simulink model "PubIfDecisionLM_MDL"  (R2020b)
settings: configuration reference "DspaceConfig" (kept outside this file)
PostLoadFcn:
  | if any(exist('dsrtsu_mdlpostloadfcn', 'file') ~= 0), dsrtsu_mdlpostloadfcn('Execute', bdroot); end
InitFcn:
  | , if any(exist('dsmpb_private', 'file') ~= 0), dsmpb_private('dsmpb_mdlclblib', 'Init', bdroot); end,
undefined symbols (not defined in the file or in its folder): OFM_OBJ_FUSIONTYPE_E, OFM_OBJ_MOVINGSTATE_E, OFM_OBJ_ORIENTATION_E, OFM_OBJ_TYPE_E, P_LM_Cyc, P_LM_EMLHistKapRcdBufSize, P_LM_EMLHistTrajBaseDis, P_LM_EMLHistTrajPNum, P_LM_EMLKapCorrMaxThre, P_LM_EMLMinKapThre, P_LM_EMLPathDisDiffThre, P_LM_EMLQuaFiltPar, P_LM_EMLTurnActKapThre, P_LM_EMLValidQuaThre, P_LM_FntPath1Disgap, P_LM_FntPath1MinDis, P_LM_FntPath1Timegap, P_LM_FntPath2Disgap, P_LM_FntPath2MinDis, P_LM_FntPath2Timegap, P_LM_FntPath3Disgap, P_LM_FntPath3MinDis, P_LM_FntPath3Timegap, P_LM_FusBLParFiltP, P_LM_FusEVDifC2Thre, P_LM_FusEVOPath1AllVSLDisThre, P_LM_FusEVOPath1AllVSLLostNumThre, P_LM_FusEVOPath1AllVSLQuaThre, P_LM_FusEVOPath1OTLFacNLC, P_LM_FusOTLQuaThre, P_LM_FusOTLSW, P_LM_FusParC0Index, P_LM_FusParC1Index, P_LM_FusParC2Index, P_LM_FusParC3Index, P_LM_FusVSLQuaThre, P_LM_FusVSLSW, P_LM_FusVSLValidSteerWheerAngThre, P_LM_FusVSLValidVxvThre, P_LM_LaneWidth, P_LM_OTLBufTPInfoEvaFactor, P_LM_OTLObjNum, P_LM_OTLObjSelectAgeThre, P_LM_OTLObjSelectDxAssessVx, P_LM_OTLObjSelectDxThre, P_LM_OTLObjSelectVxThre, P_LM_OTLObjSelectVyAssessDx, P_LM_OTLObjSelectVyThre, P_LM_OTLTrajPntBaseDis, P_LM_OTLTrajStdThre, P_LM_VSLAvailLineNum, P_LM_VSLBLSDiffThre, P_LM_VSLBLSDisRatio, P_LM_VSLFusBLParFiltP_C1, P_LM_VSLFusBLParFiltP_C2, P_LM_VSLFusBLParFiltP_C3, P_LM_VSLFusBLParFiltP_Quality, P_LM_VSLHistTrajBaseDis, P_LM_VSLHistTrajPNum, P_LM_VSLLCC0diff ... (+18)
libraries: simulink x145, LM_LIB x43
(part 18 of 24)

== system PubIfDecisionLM_MDL/Subsystem2/LM_OTL/LM_OTL_MovObjTrajRecord3/LM_OTL_MovObjSelc/LM_OTL_MovObjInterestedSelc/LM_OTL_ObjSelcIndexCheck/RigObj1Check/If Action Subsystem1 ==
  RigObj1CheckInfo : Inport
  LM_OTL_MovObjValid : Inport  Port=2
  Object_DX : Inport  Port=3
  Action Port : ActionPort  ActionPortLabel=else
  Compare To Constant1 : simulink/Logic and Bit Operations/Compare To Constant  relop=<=  const=-1.45  OutDataTypeStr=boolean
  Compare To Constant2 : simulink/Logic and Bit Operations/Compare To Constant  relop=>  const=-6  OutDataTypeStr=boolean
  Constant : Constant  Value=0  OutDataTypeStr=int32
  Logical Operator : Logic  AllPortsSameDT=off  OutDataTypeStr=boolean
  Logical Operator1 : Logic  AllPortsSameDT=off  OutDataTypeStr=boolean
  Multiport Switch : MultiPortSwitch  Inputs=1
  Multiport Switch1 : MultiPortSwitch  Inputs=1
  Switch : Switch  Criteria=u2 > Threshold
  LM_OTLRigObj1Index : Outport
  wires:
  Logical Operator1/1 -> Logical Operator/2
  Logical Operator/1 -> Switch/2
  Multiport Switch1/1 -> Compare To Constant2/1, Compare To Constant1/1
  Compare To Constant1/1 -> Logical Operator1/1
  Compare To Constant2/1 -> Logical Operator1/2
  Object_DX/1 -> Multiport Switch1/2
  LM_OTL_MovObjValid/1 -> Multiport Switch/2
  RigObj1CheckInfo/1 -> Multiport Switch1/1, Multiport Switch/1, Switch/1
  Switch/1 -> LM_OTLRigObj1Index/1
  Constant/1 -> Switch/3
  Multiport Switch/1 -> Logical Operator/1

== system PubIfDecisionLM_MDL/Subsystem2/LM_OTL/LM_OTL_MovObjTrajRecord3/LM_OTL_MovObjSelc/LM_OTL_MovObjInterestedSelc/LM_OTL_ObjSelcIndexCheck/RigObj2Check/If Action Subsystem ==
  Action Port : ActionPort  ActionPortLabel=if(u1 == 0)
  Constant : Constant  Value=0  OutDataTypeStr=int32
  LM_OTLLeObj1Index : Outport
  wires:
  Constant/1 -> LM_OTLLeObj1Index/1

== system PubIfDecisionLM_MDL/Subsystem2/LM_OTL/LM_OTL_MovObjTrajRecord3/LM_OTL_MovObjSelc/LM_OTL_MovObjInterestedSelc/LM_OTL_ObjSelcIndexCheck/RigObj2Check/If Action Subsystem1 ==
  RigObj2CheckInfo : Inport
  LM_OTL_MovObjValid : Inport  Port=2
  Object_DX : Inport  Port=3
  Action Port : ActionPort  ActionPortLabel=else
  Compare To Constant1 : simulink/Logic and Bit Operations/Compare To Constant  relop=<=  const=-2  OutDataTypeStr=boolean
  Compare To Constant2 : simulink/Logic and Bit Operations/Compare To Constant  relop=>  const=-6  OutDataTypeStr=boolean
  Constant : Constant  Value=0  OutDataTypeStr=int32
  Logical Operator : Logic  AllPortsSameDT=off  OutDataTypeStr=boolean
  Logical Operator1 : Logic  AllPortsSameDT=off  OutDataTypeStr=boolean
  Multiport Switch : MultiPortSwitch  Inputs=1
  Multiport Switch1 : MultiPortSwitch  Inputs=1
  Switch : Switch  Criteria=u2 > Threshold
  LM_OTLRigObj2Index : Outport
  wires:
  Logical Operator1/1 -> Logical Operator/2
  Logical Operator/1 -> Switch/2
  Multiport Switch1/1 -> Compare To Constant2/1, Compare To Constant1/1
  Compare To Constant1/1 -> Logical Operator1/1
  Compare To Constant2/1 -> Logical Operator1/2
  Object_DX/1 -> Multiport Switch1/2
  LM_OTL_MovObjValid/1 -> Multiport Switch/2
  RigObj2CheckInfo/1 -> Multiport Switch1/1, Multiport Switch/1, Switch/1
  Switch/1 -> LM_OTLRigObj2Index/1
  Constant/1 -> Switch/3
  Multiport Switch/1 -> Logical Operator/1

== system PubIfDecisionLM_MDL/Subsystem2/LM_OTL/LM_OTL_MovObjTrajRecord3/LM_OTL_MovObjSelc/Subsystem3/LM_OTL_MovObjSelect/LM_OTL_ExistProbAssess/MultiRader ==
  Action Port : ActionPort  ActionPortLabel=elseif((u1==6|u1==10|u1==12|u1==14))
  Constant : Constant  Value=0.5
  Out1 : Outport
  wires:
  Constant/1 -> Out1/1

== system PubIfDecisionLM_MDL/Subsystem2/LM_OTL/LM_OTL_MovObjTrajRecord3/LM_OTL_MovObjSelc/Subsystem3/LM_OTL_MovObjSelect/LM_OTL_ExistProbAssess/Rader&Video ==
  Action Port : ActionPort  ActionPortLabel=elseif((u1==3|u1==5|u1==7|u1==9|u1==11|u1==13|u1==15))
  Constant : Constant  Value=0.4
  Out1 : Outport
  wires:
  Constant/1 -> Out1/1

== system PubIfDecisionLM_MDL/Subsystem2/LM_OTL/LM_OTL_MovObjTrajRecord3/LM_OTL_MovObjSelc/Subsystem3/LM_OTL_MovObjSelect/LM_OTL_ExistProbAssess/Rader&Video1 ==
  Action Port : ActionPort  ActionPortLabel=else
  Constant : Constant  Value=0
  Out1 : Outport
  wires:
  Constant/1 -> Out1/1

== system PubIfDecisionLM_MDL/Subsystem2/LM_OTL/LM_OTL_MovObjTrajRecord3/LM_OTL_MovObjSelc/Subsystem3/LM_OTL_MovObjSelect/LM_OTL_ExistProbAssess/SingleRader ==
  Action Port : ActionPort  ActionPortLabel=if(u1==2|u1==4|u1==8)
  Constant : Constant  Value=0.6
  Out1 : Outport
  wires:
  Constant/1 -> Out1/1

== system PubIfDecisionLM_MDL/Subsystem2/LM_OTL/LM_OTL_MovObjTrajRecord3/LM_OTL_ObjStoreInfoCalc/LM_OTL_BufLe1InfoUpdate1/LM_OTL_BufLe1StoreInfoCalc/LM_OTL_ObjSICCurLeObj1InBufLe1/LM_OTL_BufL1DxInfo ==
  LM_OTLCurLeLaObj1Dx : Inport
  LM_OTLCurLeLaObj1RcdFlg : Inport  Port=2
  Constant : Constant  Value=0  OutDataTypeStr=single
  Switch4 : Switch  Criteria=u2 ~= 0
  LM_OTLBufL1Objdx : Outport
  wires:
  LM_OTLCurLeLaObj1Dx/1 -> Switch4/1
  LM_OTLCurLeLaObj1RcdFlg/1 -> Switch4/2
  Switch4/1 -> LM_OTLBufL1Objdx/1  "LM_OTLBufL1Objdx"
  Constant/1 -> Switch4/3

== system PubIfDecisionLM_MDL/Subsystem2/LM_OTL/LM_OTL_MovObjTrajRecord3/LM_OTL_ObjStoreInfoCalc/LM_OTL_BufLe1InfoUpdate1/LM_OTL_BufLe1StoreInfoCalc/LM_OTL_ObjSICCurLeObj1InBufLe1/LM_OTL_BufL1DyInfo ==
  LM_OTLCurLeLaObj1Dy : Inport
  LM_OTLCurLeLaObj1RcdFlg : Inport  Port=2
  Constant : Constant  Value=0  OutDataTypeStr=single
  Switch4 : Switch  Criteria=u2 ~= 0
  LM_OTLBufL1ObjDy : Outport
  wires:
  Constant/1 -> Switch4/3
  Switch4/1 -> LM_OTLBufL1ObjDy/1  "LM_OTLBufL1ObjDy"
  LM_OTLCurLeLaObj1Dy/1 -> Switch4/1
  LM_OTLCurLeLaObj1RcdFlg/1 -> Switch4/2

== system PubIfDecisionLM_MDL/Subsystem2/LM_OTL/LM_OTL_MovObjTrajRecord3/LM_OTL_ObjStoreInfoCalc/LM_OTL_BufLe1InfoUpdate1/LM_OTL_BufLe1StoreInfoCalc/LM_OTL_ObjSICCurLeObj1InBufLe1/LM_OTL_BufL1EPInfo ==
  note: P_LM_OTLTPNum
  LM_OTLCurLeLaObj1RcdFlg : Inport
  LM_OTLBufL1EPPosK1 : Inport  Port=2
  Add : Sum
  Constant : Constant  OutDataTypeStr=uint8
  Constant1 : Constant  Value=80  OutDataTypeStr=uint8
  Constant2 : Constant  OutDataTypeStr=uint8
  Relational Operator : RelationalOperator  Operator=>  OutDataTypeStr=boolean  RndMeth=Simplest
  Switch1 : Switch  Criteria=u2 ~= 0
  Switch4 : Switch  Criteria=u2 ~= 0
  LM_OTLBufL1EPPos : Outport
  wires:
  Constant/1 -> Add/2
  LM_OTLCurLeLaObj1RcdFlg/1 -> Switch4/2
  LM_OTLBufL1EPPosK1/1 -> Switch4/3, Add/1
  Switch4/1 -> LM_OTLBufL1EPPos/1  "LM_OTLBufL1EPPos"
  Switch1/1 -> Switch4/1
  Relational Operator/1 -> Switch1/2
  Add/1 -> Switch1/3, Relational Operator/1
  Constant1/1 -> Relational Operator/2
  Constant2/1 -> Switch1/1

== system PubIfDecisionLM_MDL/Subsystem2/LM_OTL/LM_OTL_MovObjTrajRecord3/LM_OTL_ObjStoreInfoCalc/LM_OTL_BufLe1InfoUpdate1/LM_OTL_BufLe1StoreInfoCalc/LM_OTL_ObjSICCurLeObj1InBufLe1/LM_OTL_BufL1IDInfo ==
  LM_OTLCurLeLaObj1ID : Inport
  Signal Conversion : SignalConversion  OverrideOpt=off
  LM_OTLBufL1ObjID : Outport
  wires:
  LM_OTLCurLeLaObj1ID/1 -> Signal Conversion/1
  Signal Conversion/1 -> LM_OTLBufL1ObjID/1  "LM_OTLBufL1ObjID"

== system PubIfDecisionLM_MDL/Subsystem2/LM_OTL/LM_OTL_MovObjTrajRecord3/LM_OTL_ObjStoreInfoCalc/LM_OTL_BufLe1InfoUpdate1/LM_OTL_BufLe1StoreInfoCalc/LM_OTL_ObjSICCurLeObj1InBufLe1/LM_OTL_BufL1PNumInfo ==
  LM_OTLBufL1PNumK1 : Inport
  LM_OTLCurLeLaObj1RcdFlg : Inport  Port=2
  Add : Sum
  Constant : Constant  OutDataTypeStr=uint8
  Saturation : Saturate  UpperLimit=80  LowerLimit=0
  Switch4 : Switch  Criteria=u2 ~= 0
  LM_OTLBufL1PNum : Outport
  wires:
  LM_OTLBufL1PNumK1/1 -> Switch4/3, Add/1
  Switch4/1 -> LM_OTLBufL1PNum/1  "LM_OTLBufL1PNum"
  LM_OTLCurLeLaObj1RcdFlg/1 -> Switch4/2
  Add/1 -> Saturation/1
  Constant/1 -> Add/2
  Saturation/1 -> Switch4/1

== system PubIfDecisionLM_MDL/Subsystem2/LM_OTL/LM_OTL_MovObjTrajRecord3/LM_OTL_ObjStoreInfoCalc/LM_OTL_BufLe1InfoUpdate1/LM_OTL_BufLe1StoreInfoCalc/LM_OTL_ObjSICCurLeObj1InBufLe1/LM_OTL_BufL1SPInfo ==
  LM_OTLBufL1SPPosK1 : Inport
  LM_OTLBufL1EPPos : Inport  Port=2
  Add : Sum
  Constant : Constant  OutDataTypeStr=uint8
  Relational Operator : RelationalOperator  Operator===  OutDataTypeStr=boolean  RndMeth=Simplest
  Switch : Switch  Criteria=u2 ~= 0
  LM_OTLBufL1SPPos : Outport
  wires:
  Constant/1 -> Add/2
  LM_OTLBufL1SPPosK1/1 -> Switch/3, Relational Operator/2
  Switch/1 -> LM_OTLBufL1SPPos/1  "LM_OTLBufL1SPPos"
  LM_OTLBufL1EPPos/1 -> Add/1, Relational Operator/1
  Relational Operator/1 -> Switch/2
  Add/1 -> Switch/1

== system PubIfDecisionLM_MDL/Subsystem2/LM_OTL/LM_OTL_MovObjTrajRecord3/LM_OTL_ObjStoreInfoCalc/LM_OTL_BufLe1InfoUpdate1/LM_OTL_BufLe1StoreInfoCalc/LM_OTL_ObjSICCurLeObj1InBufLe1/LM_OTL_BufL1UpdateFlg ==
  LM_OTLCurLeLaObj1RcdFlg : Inport
  Signal Conversion : SignalConversion  OverrideOpt=off
  LM_OTLBufL1UpdateFlg : Outport
  wires:
  LM_OTLCurLeLaObj1RcdFlg/1 -> Signal Conversion/1
  Signal Conversion/1 -> LM_OTLBufL1UpdateFlg/1  "LM_OTLBufL1UpdateFlg"

== system PubIfDecisionLM_MDL/Subsystem2/LM_OTL/LM_OTL_MovObjTrajRecord3/LM_OTL_ObjStoreInfoCalc/LM_OTL_BufLe1InfoUpdate1/LM_OTL_BufLe1StoreInfoCalc/LM_OTL_ObjSICCurLeObj2InBufLe1/LM_OTL_BufL1DxInfo ==
  LM_OTLCurLeLaObj1Dx : Inport
  LM_OTLCurLeLaObj1RcdFlg : Inport  Port=2
  Constant : Constant  Value=0  OutDataTypeStr=single
  Switch4 : Switch  Criteria=u2 ~= 0
  LM_OTLBufL1Objdx : Outport
  wires:
  LM_OTLCurLeLaObj1Dx/1 -> Switch4/1
  LM_OTLCurLeLaObj1RcdFlg/1 -> Switch4/2
  Switch4/1 -> LM_OTLBufL1Objdx/1  "LM_OTLBufL1Objdx"
  Constant/1 -> Switch4/3

== system PubIfDecisionLM_MDL/Subsystem2/LM_OTL/LM_OTL_MovObjTrajRecord3/LM_OTL_ObjStoreInfoCalc/LM_OTL_BufLe1InfoUpdate1/LM_OTL_BufLe1StoreInfoCalc/LM_OTL_ObjSICCurLeObj2InBufLe1/LM_OTL_BufL1DyInfo ==
  LM_OTLCurLeLaObj1Dy : Inport
  LM_OTLCurLeLaObj1RcdFlg : Inport  Port=2
  Constant : Constant  Value=0  OutDataTypeStr=single
  Switch4 : Switch  Criteria=u2 ~= 0
  LM_OTLBufL1ObjDy : Outport
  wires:
  Constant/1 -> Switch4/3
  Switch4/1 -> LM_OTLBufL1ObjDy/1  "LM_OTLBufL1ObjDy"
  LM_OTLCurLeLaObj1Dy/1 -> Switch4/1
  LM_OTLCurLeLaObj1RcdFlg/1 -> Switch4/2

== system PubIfDecisionLM_MDL/Subsystem2/LM_OTL/LM_OTL_MovObjTrajRecord3/LM_OTL_ObjStoreInfoCalc/LM_OTL_BufLe1InfoUpdate1/LM_OTL_BufLe1StoreInfoCalc/LM_OTL_ObjSICCurLeObj2InBufLe1/LM_OTL_BufL1EPInfo ==
  note: P_LM_OTLTPNum
  LM_OTLCurLeLaObj1RcdFlg : Inport
  LM_OTLBufL1EPPosK1 : Inport  Port=2
  Add : Sum
  Constant : Constant  OutDataTypeStr=uint8
  Constant1 : Constant  Value=80  OutDataTypeStr=uint8
  Constant2 : Constant  OutDataTypeStr=uint8
  Relational Operator : RelationalOperator  Operator=>  OutDataTypeStr=boolean  RndMeth=Simplest
  Switch1 : Switch  Criteria=u2 ~= 0
  Switch4 : Switch  Criteria=u2 ~= 0
  LM_OTLBufL1EPPos : Outport
  wires:
  Constant/1 -> Add/2
  LM_OTLCurLeLaObj1RcdFlg/1 -> Switch4/2
  LM_OTLBufL1EPPosK1/1 -> Switch4/3, Add/1
  Switch4/1 -> LM_OTLBufL1EPPos/1  "LM_OTLBufL1EPPos"
  Switch1/1 -> Switch4/1
  Relational Operator/1 -> Switch1/2
  Add/1 -> Switch1/3, Relational Operator/1
  Constant1/1 -> Relational Operator/2
  Constant2/1 -> Switch1/1

== system PubIfDecisionLM_MDL/Subsystem2/LM_OTL/LM_OTL_MovObjTrajRecord3/LM_OTL_ObjStoreInfoCalc/LM_OTL_BufLe1InfoUpdate1/LM_OTL_BufLe1StoreInfoCalc/LM_OTL_ObjSICCurLeObj2InBufLe1/LM_OTL_BufL1IDInfo ==
  LM_OTLCurLeLaObj1ID : Inport
  Signal Conversion : SignalConversion  OverrideOpt=off
  LM_OTLBufL1ObjID : Outport
  wires:
  LM_OTLCurLeLaObj1ID/1 -> Signal Conversion/1
  Signal Conversion/1 -> LM_OTLBufL1ObjID/1  "LM_OTLBufL1ObjID"

== system PubIfDecisionLM_MDL/Subsystem2/LM_OTL/LM_OTL_MovObjTrajRecord3/LM_OTL_ObjStoreInfoCalc/LM_OTL_BufLe1InfoUpdate1/LM_OTL_BufLe1StoreInfoCalc/LM_OTL_ObjSICCurLeObj2InBufLe1/LM_OTL_BufL1PNumInfo ==
  LM_OTLBufL1PNumK1 : Inport
  LM_OTLCurLeLaObj1RcdFlg : Inport  Port=2
  Add : Sum
  Constant : Constant  OutDataTypeStr=uint8
  Saturation : Saturate  UpperLimit=80  LowerLimit=0
  Switch4 : Switch  Criteria=u2 ~= 0
  LM_OTLBufL1PNum : Outport
  wires:
  LM_OTLBufL1PNumK1/1 -> Switch4/3, Add/1
  Switch4/1 -> LM_OTLBufL1PNum/1  "LM_OTLBufL1PNum"
  LM_OTLCurLeLaObj1RcdFlg/1 -> Switch4/2
  Add/1 -> Saturation/1
  Constant/1 -> Add/2
  Saturation/1 -> Switch4/1

== system PubIfDecisionLM_MDL/Subsystem2/LM_OTL/LM_OTL_MovObjTrajRecord3/LM_OTL_ObjStoreInfoCalc/LM_OTL_BufLe1InfoUpdate1/LM_OTL_BufLe1StoreInfoCalc/LM_OTL_ObjSICCurLeObj2InBufLe1/LM_OTL_BufL1SPInfo ==
  LM_OTLBufL1SPPosK1 : Inport
  LM_OTLBufL1EPPos : Inport  Port=2
  Add : Sum
  Constant : Constant  OutDataTypeStr=uint8
  Relational Operator : RelationalOperator  Operator===  OutDataTypeStr=boolean  RndMeth=Simplest
  Switch : Switch  Criteria=u2 ~= 0
  LM_OTLBufL1SPPos : Outport
  wires:
  Constant/1 -> Add/2
  LM_OTLBufL1SPPosK1/1 -> Switch/3, Relational Operator/2
  Switch/1 -> LM_OTLBufL1SPPos/1  "LM_OTLBufL1SPPos"
  LM_OTLBufL1EPPos/1 -> Add/1, Relational Operator/1
  Relational Operator/1 -> Switch/2
  Add/1 -> Switch/1

== system PubIfDecisionLM_MDL/Subsystem2/LM_OTL/LM_OTL_MovObjTrajRecord3/LM_OTL_ObjStoreInfoCalc/LM_OTL_BufLe1InfoUpdate1/LM_OTL_BufLe1StoreInfoCalc/LM_OTL_ObjSICCurLeObj2InBufLe1/LM_OTL_BufL1UpdateFlg ==
  LM_OTLCurLeLaObj1RcdFlg : Inport
  Signal Conversion : SignalConversion  OverrideOpt=off
  LM_OTLBufL1UpdateFlg : Outport
  wires:
  LM_OTLCurLeLaObj1RcdFlg/1 -> Signal Conversion/1
  Signal Conversion/1 -> LM_OTLBufL1UpdateFlg/1  "LM_OTLBufL1UpdateFlg"

== system PubIfDecisionLM_MDL/Subsystem2/LM_OTL/LM_OTL_MovObjTrajRecord3/LM_OTL_ObjStoreInfoCalc/LM_OTL_BufLe1InfoUpdate1/LM_OTL_BufLe1StoreInfoCalc/LM_OTL_ObjSICNoCurObjInBufLe1/LM_OTL_BufL1DxInfo ==
  LM_OTLCurLeLaObj1Index : Inport
  LM_OTLCurLeLaObj2Index : Inport  Port=2
  LM_OTLCurLeLaObj1RcdedFlg : Inport  Port=3
  LM_OTLCurLeLaObj1Dx : Inport  Port=4
  LM_OTLCurLeLaObj2Dx : Inport  Port=5
  Compare To Zero : simulink/Logic and Bit Operations/Compare To Zero  relop===  OutDataTypeStr=boolean
  Compare To Zero1 : simulink/Logic and Bit Operations/Compare To Zero  relop===  OutDataTypeStr=boolean
  Compare To Zero2 : simulink/Logic and Bit Operations/Compare To Zero  relop===  OutDataTypeStr=boolean
  Constant : Constant  Value=0  OutDataTypeStr=single
  Constant1 : Constant  Value=0  OutDataTypeStr=single
  DocBlock : simulink/Model-Wide Utilities/DocBlock  DocumentType=Text
      content=|
      | 1. 功能描述
      |    该模块主要功能
      | 2. 算法说明
      | 2.1 当左车道最近目标索引为0时，即左车道无目标，输出0
      | 2.2 当左车道最近目标索引不为0时
      |     2.2.1 如果左车道最近目标ID未在buffer中存储，则输出左车道最近目标的dx
      |     2.2.2 如果左车道最近目标ID已经在buffer中存储
      |           2.2.2.1 如果左车道第二近目标ID不为0，则输出左车道第二近目标dx
      |           2.2.2.2 如果左车道第二近目标ID为0，则输出0
  Switch1 : Switch  Criteria=u2 ~= 0
  Switch2 : Switch  Criteria=u2 ~= 0
  Switch4 : Switch  Criteria=u2 ~= 0
  LM_OTLBufL1Objdx : Outport
  wires:
  LM_OTLCurLeLaObj1RcdedFlg/1 -> Compare To Zero1/1
  Switch1/1 -> Switch4/3
  Switch4/1 -> LM_OTLBufL1Objdx/1  "LM_OTLBufL1Objdx"
  LM_OTLCurLeLaObj1Index/1 -> Compare To Zero/1
  LM_OTLCurLeLaObj2Index/1 -> Compare To Zero2/1
  Compare To Zero/1 -> Switch4/2
  Constant/1 -> Switch4/1
  Compare To Zero1/1 -> Switch1/2
  LM_OTLCurLeLaObj1Dx/1 -> Switch1/1
  Compare To Zero2/1 -> Switch2/2
  Constant1/1 -> Switch2/1
  Switch2/1 -> Switch1/3
  LM_OTLCurLeLaObj2Dx/1 -> Switch2/3

== system PubIfDecisionLM_MDL/Subsystem2/LM_OTL/LM_OTL_MovObjTrajRecord3/LM_OTL_ObjStoreInfoCalc/LM_OTL_BufLe1InfoUpdate1/LM_OTL_BufLe1StoreInfoCalc/LM_OTL_ObjSICNoCurObjInBufLe1/LM_OTL_BufL1DyInfo ==
  LM_OTLCurLeLaObj1Index : Inport
  LM_OTLCurLeLaObj2Index : Inport  Port=2
  LM_OTLCurLeLaObj1RcdedFlg : Inport  Port=3
  LM_OTLCurLeLaObj1Dy : Inport  Port=4
  LM_OTLCurLeLaObj2Dy : Inport  Port=5
  Compare To Zero : simulink/Logic and Bit Operations/Compare To Zero  relop===  OutDataTypeStr=boolean
  Compare To Zero1 : simulink/Logic and Bit Operations/Compare To Zero  relop===  OutDataTypeStr=boolean
  Compare To Zero2 : simulink/Logic and Bit Operations/Compare To Zero  relop===  OutDataTypeStr=boolean
  Constant : Constant  Value=0  OutDataTypeStr=single
  Constant1 : Constant  Value=0  OutDataTypeStr=single
  Switch1 : Switch  Criteria=u2 ~= 0
  Switch2 : Switch  Criteria=u2 ~= 0
  Switch4 : Switch  Criteria=u2 ~= 0
  LM_OTLBufL1Objdy : Outport
  wires:
  Constant/1 -> Switch4/1
  LM_OTLCurLeLaObj1Dy/1 -> Switch1/1
  Compare To Zero1/1 -> Switch1/2
  LM_OTLCurLeLaObj1Index/1 -> Compare To Zero/1
  Switch1/1 -> Switch4/3
  Switch4/1 -> LM_OTLBufL1Objdy/1  "LM_OTLBufL1Objdy"
  Compare To Zero/1 -> Switch4/2
  Constant1/1 -> Switch2/1
  LM_OTLCurLeLaObj1RcdedFlg/1 -> Compare To Zero1/1
  LM_OTLCurLeLaObj2Index/1 -> Compare To Zero2/1
  LM_OTLCurLeLaObj2Dy/1 -> Switch2/3
  Compare To Zero2/1 -> Switch2/2
  Switch2/1 -> Switch1/3

== system PubIfDecisionLM_MDL/Subsystem2/LM_OTL/LM_OTL_MovObjTrajRecord3/LM_OTL_ObjStoreInfoCalc/LM_OTL_BufLe1InfoUpdate1/LM_OTL_BufLe1StoreInfoCalc/LM_OTL_ObjSICNoCurObjInBufLe1/LM_OTL_BufL1EPInfo ==
  LM_OTLBufL1SPPos : Inport
  Signal Conversion : SignalConversion  OverrideOpt=off
  LM_OTLBufL1EPPos : Outport
  wires:
  Signal Conversion/1 -> LM_OTLBufL1EPPos/1  "LM_OTLBufL1EPPos"
  LM_OTLBufL1SPPos/1 -> Signal Conversion/1

== system PubIfDecisionLM_MDL/Subsystem2/LM_OTL/LM_OTL_MovObjTrajRecord3/LM_OTL_ObjStoreInfoCalc/LM_OTL_BufLe1InfoUpdate1/LM_OTL_BufLe1StoreInfoCalc/LM_OTL_ObjSICNoCurObjInBufLe1/LM_OTL_BufL1IDInfo ==
  LM_OTLCurLeLaObj1Index : Inport
  LM_OTLCurLeLaObj2Index : Inport  Port=2
  LM_OTLCurLeLaObj1RcdedFlg : Inport  Port=3
  LM_OTLCurLeLaObj1ID : Inport  Port=4
  LM_OTLCurLeLaObj2ID : Inport  Port=5
  Compare To Zero : simulink/Logic and Bit Operations/Compare To Zero  relop===  OutDataTypeStr=boolean
  Compare To Zero1 : simulink/Logic and Bit Operations/Compare To Zero  relop===  OutDataTypeStr=boolean
  Compare To Zero2 : simulink/Logic and Bit Operations/Compare To Zero  relop===  OutDataTypeStr=boolean
  Compare To Zero3 : simulink/Logic and Bit Operations/Compare To Zero  relop=~=  OutDataTypeStr=boolean
  Constant : Constant  Value=0  OutDataTypeStr=single
  Constant1 : Constant  Value=0  OutDataTypeStr=single
  Switch1 : Switch  Criteria=u2 ~= 0
  Switch2 : Switch  Criteria=u2 ~= 0
  Switch4 : Switch  Criteria=u2 ~= 0
  LM_OTLBufL1UpdateFlg : Outport
  LM_OTLBufL1ObjID : Outport  Port=2
  wires:
  Constant/1 -> Switch4/1
  LM_OTLCurLeLaObj1ID/1 -> Switch1/1
  Compare To Zero1/1 -> Switch1/2
  LM_OTLCurLeLaObj1Index/1 -> Compare To Zero/1
  Switch1/1 -> Switch4/3
  Switch4/1 -> Compare To Zero3/1, LM_OTLBufL1ObjID/1  "LM_OTLBufL1ObjID"
  Compare To Zero/1 -> Switch4/2
  Constant1/1 -> Switch2/1
  LM_OTLCurLeLaObj1RcdedFlg/1 -> Compare To Zero1/1
  LM_OTLCurLeLaObj2Index/1 -> Compare To Zero2/1
  LM_OTLCurLeLaObj2ID/1 -> Switch2/3
  Compare To Zero2/1 -> Switch2/2
  Switch2/1 -> Switch1/3
  Compare To Zero3/1 -> LM_OTLBufL1UpdateFlg/1

== system PubIfDecisionLM_MDL/Subsystem2/LM_OTL/LM_OTL_MovObjTrajRecord3/LM_OTL_ObjStoreInfoCalc/LM_OTL_BufLe1InfoUpdate1/LM_OTL_BufLe1StoreInfoCalc/LM_OTL_ObjSICNoCurObjInBufLe1/LM_OTL_BufL1PNumInfo ==
  LM_OTLCurLeLaObj1Index : Inport
  LM_OTLCurLeLaObj2Index : Inport  Port=2
  LM_OTLCurLeLaObj1RcdedFlg : Inport  Port=3
  Compare To Zero : simulink/Logic and Bit Operations/Compare To Zero  relop===  OutDataTypeStr=boolean
  Compare To Zero1 : simulink/Logic and Bit Operations/Compare To Zero  relop===  OutDataTypeStr=boolean
  Compare To Zero2 : simulink/Logic and Bit Operations/Compare To Zero  relop===  OutDataTypeStr=boolean
  Constant : Constant  Value=0  OutDataTypeStr=uint8
  Constant1 : Constant  Value=0  OutDataTypeStr=uint8
  Constant2 : Constant  OutDataTypeStr=uint8
  Constant3 : Constant  OutDataTypeStr=uint8
  Switch1 : Switch  Criteria=u2 ~= 0
  Switch2 : Switch  Criteria=u2 ~= 0
  Switch4 : Switch  Criteria=u2 ~= 0
  LM_OTLBufL1TPNum : Outport
  wires:
  Switch2/1 -> Switch1/3
  Switch4/1 -> LM_OTLBufL1TPNum/1  "LM_OTLBufL1TPNum"
  Compare To Zero2/1 -> Switch2/2
  Switch1/1 -> Switch4/3
  LM_OTLCurLeLaObj1RcdedFlg/1 -> Compare To Zero1/1
  LM_OTLCurLeLaObj2Index/1 -> Compare To Zero2/1
  LM_OTLCurLeLaObj1Index/1 -> Compare To Zero/1
  Constant1/1 -> Switch2/1
  Compare To Zero1/1 -> Switch1/2
  Constant/1 -> Switch4/1
  Compare To Zero/1 -> Switch4/2
  Constant2/1 -> Switch1/1
  Constant3/1 -> Switch2/3

== system PubIfDecisionLM_MDL/Subsystem2/LM_OTL/LM_OTL_MovObjTrajRecord3/LM_OTL_ObjStoreInfoCalc/LM_OTL_BufLe1InfoUpdate1/LM_OTL_BufLe1StoreInfoCalc/LM_OTL_ObjSICNoCurObjInBufLe1/LM_OTL_BufL1SPInfo ==
  LM_OTLCurLeLaObj1Index : Inport
  LM_OTLCurLeLaObj2Index : Inport  Port=2
  LM_OTLCurLeLaObj1RcdedFlg : Inport  Port=3
  LM_OTLBufL1LastTPValid : Inport  Port=4
  LM_OTLBufL1LastEPPos : Inport  Port=5
  Add : Sum
  Compare To Zero{,1..3} (4 alike) : simulink/Logic and Bit Operations/Compare To Zero  relop===  OutDataTypeStr=boolean
  Constant : Constant  Value=0  OutDataTypeStr=uint8
  Constant1 : Constant  Value=0  OutDataTypeStr=uint8
  Constant2 : Constant  OutDataTypeStr=uint8
  Switch{,1..2,4} (4 alike) : Switch  Criteria=u2 ~= 0
  LM_OTLBufL1SPPos : Outport
  wires:
  Constant/1 -> Switch4/1
  Compare To Zero/1 -> Switch4/2
  Constant1/1 -> Switch2/1
  Compare To Zero1/1 -> Switch1/2
  LM_OTLCurLeLaObj2Index/1 -> Compare To Zero2/1
  Switch1/1 -> Switch4/3
  LM_OTLCurLeLaObj1RcdedFlg/1 -> Compare To Zero1/1
  LM_OTLCurLeLaObj1Index/1 -> Compare To Zero/1
  Compare To Zero2/1 -> Switch2/2
  Switch4/1 -> LM_OTLBufL1SPPos/1  "LM_OTLBufL1SPPos"
  Switch/1 -> Switch1/1
  Switch2/1 -> Switch1/3
  Add/1 -> Switch2/3, Switch/3
  LM_OTLBufL1LastTPValid/1 -> Compare To Zero3/1
  Compare To Zero3/1 -> Switch/2
  Constant2/1 -> Add/2, Switch/1
  LM_OTLBufL1LastEPPos/1 -> Add/1

== system PubIfDecisionLM_MDL/Subsystem2/LM_VSL/LM_VSLFntPath/LM_VSL_LineInfoEvalutaion/LM_VSL_BaseLinePCalc3/Subsystem/Switch Case Action Subsystem/LM_VSLBaseParCalc ==
  LM_VSLLineQualitySum : Inport
  Diffnum : Inport  Port=2
  LM_VSLLineMinQualityIndex : Inport  Port=3
  LM_VSLLineQualityVect : Inport  Port=4
  LM_VSLMinQualityLineValid : Inport  Port=5
  LM_VSLLineC1Vect : Inport  Port=6
  LM_VSLLineC2Vect : Inport  Port=7
  LM_VSLLineC3Vect : Inport  Port=8
  1-D Lookup Table1 : Lookup_n-D  NumberOfTableDimensions=1  BreakpointsForDimension1=P_LM_VSLAvailLineNum  Table=P_LM_VSLLineBaseQualityRatio  InternalRulePriority=Speed  RndMeth=Simplest  InputSameDT=on
  Add{,1..3} (4 alike) : Sum
  Compare To Zero : simulink/Logic and Bit Operations/Compare To Zero  relop===  OutDataTypeStr=boolean
  Constant : Constant  OutDataTypeStr=single
  Constant1 : Constant  Value=0  OutDataTypeStr=single
  Constant2 : Constant  OutDataTypeStr=uint8
  Divide : Product  Inputs=*/
  For Iterator : ForIterator  IterationLimit=4
  Index Vector{,1..3} (4 alike) : MultiPortSwitch  Inputs=1
  Product{,1..4} (5 alike) : Product
  Relational Operator1 : RelationalOperator  Operator===  OutDataTypeStr=boolean  RndMeth=Nearest
  Relational Operator2 : RelationalOperator  Operator===  OutDataTypeStr=boolean  RndMeth=Nearest
  Switch{,1..5,8} (7 alike) : Switch  Criteria=u2 ~= 0
  Unit Delay{,1..3} (4 alike) : UnitDelay  SampleTime=-1  HasFrameUpgradeWarning=on
  LM_VSLBaseC1 : Outport
  LM_VSLBaseC2 : Outport  Port=2
  LM_VSLBaseC3 : Outport  Port=3
  LM_VSLBaseQuality : Outport  Port=4
  wires:
  Diffnum/1 -> 1-D Lookup Table1/1
  Product4/1 -> LM_VSLBaseQuality/1
  1-D Lookup Table1/1 -> Product4/1
  Constant1/1 -> Switch4/3
  LM_VSLMinQualityLineValid/1 -> Switch4/2
  Index Vector2/1 -> Product1/1
  Add2/1 -> Switch3/3
  Unit Delay2/1 -> Add2/2
  Product2/1 -> Add2/1, Switch3/1
  Switch3/1 -> LM_VSLBaseC3/1, Unit Delay2/1
  Switch2/1 -> Unit Delay1/1, LM_VSLBaseC2/1
  Product1/1 -> Switch2/1, Add1/1
  Unit Delay1/1 -> Add1/2
  Add1/1 -> Switch2/3
  LM_VSLLineC2Vect/1 -> Index Vector2/2
  LM_VSLLineC3Vect/1 -> Index Vector3/2
  Index Vector1/1 -> Product/2
  LM_VSLLineC1Vect/1 -> Index Vector1/2
  Add/1 -> Switch/3
  Unit Delay/1 -> Add/2
  Product/1 -> Add/1, Switch/1
  Switch/1 -> LM_VSLBaseC1/1, Unit Delay/1
  Constant2/1 -> Relational Operator2/2
  LM_VSLLineQualitySum/1 -> Switch5/3, Compare To Zero/1
  For Iterator/1 -> Index Vector/1, Index Vector3/1, Index Vector2/1, Index Vector1/1, Relational Operator1/2, Relational Operator2/1
  LM_VSLLineMinQualityIndex/1 -> Relational Operator1/1
  Relational Operator1/1 -> Switch1/2
  LM_VSLLineQualityVect/1 -> Index Vector/2
  Index Vector/1 -> Switch1/3, Switch4/1
  Switch4/1 -> Switch1/1
  Index Vector3/1 -> Product2/2
  Switch5/1 -> Divide/2
  Compare To Zero/1 -> Switch5/2
  Constant/1 -> Switch5/1
  Unit Delay3/1 -> Add3/2
  Switch1/1 -> Product3/1, Divide/1
  Divide/1 -> Product3/2, Product/1, Product2/1, Product1/2
  Add3/1 -> Switch8/3
  Switch8/1 -> Unit Delay3/1, Product4/2
  Relational Operator2/1 -> Switch8/2, Switch3/2, Switch2/2, Switch/2
  Product3/1 -> Add3/1, Switch8/1

== system PubIfDecisionLM_MDL/Subsystem2/LM_VSL/LM_VSLFntPath/LM_VSL_LineInfoEvalutaion/LM_VSL_BaseLinePCalc3/Subsystem/Switch Case Action Subsystem/LM_VSLLineQualitySumCalc ==
  LM_VSLLineMinQualityIndex : Inport
  LM_VSLLineQualityVect : Inport  Port=2
  LM_VSLMinQualityLineValid : Inport  Port=3
  LM_VSLLineDisFntVect : Inport  Port=4
  LM_VSLBLFntDis : Inport  Port=5
  Add : Sum
  Constant : Constant
  Constant1 : Constant  OutDataTypeStr=single
  Constant2 : Constant  Value=0  OutDataTypeStr=single
  Constant3 : Constant  Value=2  OutDataTypeStr=single
  For Iterator : ForIterator  IterationLimit=4
  Index Vector : MultiPortSwitch  Inputs=1
  Index Vector1 : MultiPortSwitch  Inputs=1
  Logical Operator : Logic  Operator=NOT  AllPortsSameDT=off  OutDataTypeStr=boolean
  Logical Operator1 : Logic  Operator=OR  AllPortsSameDT=off  OutDataTypeStr=boolean
  Relational Operator : RelationalOperator  Operator===  OutDataTypeStr=boolean  RndMeth=Nearest
  Relational Operator1 : RelationalOperator  Operator===  OutDataTypeStr=boolean  RndMeth=Nearest
  Subsystem : Subsystem
  Switch{,1..3} (4 alike) : Switch  Criteria=u2 ~= 0
  Unit Delay : UnitDelay  SampleTime=-1  HasFrameUpgradeWarning=on
  LM_VSLLineQualitySum : Outport
  Diffnum : Outport  Port=2
  wires:
  Switch3/1 -> Diffnum/1
  Constant3/1 -> Switch3/3
  Constant1/1 -> Switch3/1
  Subsystem/1(LM_VSLFntDisValid) -> Logical Operator1/1
  LM_VSLBLFntDis/1 -> Subsystem/2(LM_VSLBLFntDis)
  Index Vector1/1 -> Subsystem/1(LM_VSLLineDisFntVect)
  Logical Operator1/1 -> Logical Operator/1
  LM_VSLMinQualityLineValid/1 -> Logical Operator1/2
  Constant2/1 -> Switch2/1
  Logical Operator/1 -> Switch2/2, Switch3/2
  Relational Operator1/1 -> Switch1/2
  LM_VSLLineDisFntVect/1 -> Index Vector1/2
  Unit Delay/1 -> Add/2
  Switch/1 -> LM_VSLLineQualitySum/1, Unit Delay/1  "LM_VSLLineQualitySum"
  Add/1 -> Switch/3
  Switch1/1 -> Switch/1, Add/1
  Switch2/1 -> Switch1/1
  Index Vector/1 -> Switch2/3, Switch1/3
  LM_VSLLineQualityVect/1 -> Index Vector/2
  LM_VSLLineMinQualityIndex/1 -> Relational Operator1/1
  Relational Operator/1 -> Switch/2
  Constant/1 -> Relational Operator/2
  For Iterator/1 -> Index Vector1/1, Index Vector/1, Relational Operator1/2, Relational Operator/1

== system PubIfDecisionLM_MDL/Subsystem2/LM_VSL/LM_VSLFntPath/LM_VSL_LineInfoEvalutaion/LM_VSL_BaseLinePCalc3/Subsystem/Switch Case Action Subsystem3/LM_VSLBaseParCalc ==
  LM_VSLLineQualitySum : Inport
  LM_VSLLineMinQualityIndex : Inport  Port=2
  LM_VSLLineQualityVect : Inport  Port=3
  LM_VSLMinQualityLineValid : Inport  Port=4
  Diffnum : Inport  Port=5
  LM_VSLDiffMaxValid : Inport  Port=6
  LM_VSLLineC1Vect : Inport  Port=7
  LM_VSLLineC2Vect : Inport  Port=8
  LM_VSLLineC3Vect : Inport  Port=9
  1-D Lookup Table : Lookup_n-D  NumberOfTableDimensions=1  BreakpointsForDimension1=P_LM_VSLAvailLineNum  Table=P_LM_VSLLineBaseQualityRatio  InternalRulePriority=Speed  RndMeth=Simplest  InputSameDT=on
  Add{,1..3} (4 alike) : Sum
  Compare To Zero : simulink/Logic and Bit Operations/Compare To Zero  relop===  OutDataTypeStr=boolean
  Constant : Constant  OutDataTypeStr=single
  Constant1 : Constant  Value=0  OutDataTypeStr=single
  Constant2 : Constant  OutDataTypeStr=uint8
  Constant3 : Constant  Value=0  OutDataTypeStr=single
  Divide : Product  Inputs=*/
  For Iterator : ForIterator  IterationLimit=4
  Index Vector{,1..4} (5 alike) : MultiPortSwitch  Inputs=1
  Logical Operator1 : Logic  Operator=NOT  AllPortsSameDT=off  OutDataTypeStr=boolean
  Product{,1..4} (5 alike) : Product
  Relational Operator1 : RelationalOperator  Operator===  OutDataTypeStr=boolean  RndMeth=Nearest
  Relational Operator2 : RelationalOperator  Operator===  OutDataTypeStr=boolean  RndMeth=Nearest
  Switch{,1..6,8} (8 alike) : Switch  Criteria=u2 ~= 0
  Unit Delay{,1..3} (4 alike) : UnitDelay  SampleTime=-1  HasFrameUpgradeWarning=on
  LM_VSLBaseC1 : Outport
  LM_VSLBaseC2 : Outport  Port=2
  LM_VSLBaseC3 : Outport  Port=3
  LM_VSLBaseQuality : Outport  Port=4
  wires:
  Product4/1 -> LM_VSLBaseQuality/1
  1-D Lookup Table/1 -> Product4/1
  Logical Operator1/1 -> Switch6/2
  Constant3/1 -> Switch6/1
  LM_VSLDiffMaxValid/1 -> Index Vector4/2
  Diffnum/1 -> 1-D Lookup Table/1
  Constant/1 -> Switch5/1
  Compare To Zero/1 -> Switch5/2
  Switch5/1 -> Divide/2
  Index Vector3/1 -> Product2/2
  Switch4/1 -> Switch1/1
  Index Vector/1 -> Switch4/1, Switch1/3
  LM_VSLLineQualityVect/1 -> Index Vector/2
  Relational Operator1/1 -> Switch1/2
  LM_VSLLineMinQualityIndex/1 -> Relational Operator1/1
  For Iterator/1 -> Relational Operator2/1, Relational Operator1/2, Index Vector1/1, Index Vector2/1, Index Vector3/1, Index Vector/1, Index Vector4/1
  Switch6/1 -> Product3/1, Divide/1
  LM_VSLLineQualitySum/1 -> Compare To Zero/1, Switch5/3
  Divide/1 -> Product1/2, Product2/1, Product3/2, Product/1
  Constant2/1 -> Relational Operator2/2
  Switch/1 -> Unit Delay/1, LM_VSLBaseC1/1
  Product/1 -> Switch/1, Add/1
  Unit Delay/1 -> Add/2
  Add/1 -> Switch/3
  LM_VSLLineC1Vect/1 -> Index Vector1/2
  Index Vector1/1 -> Product/2
  LM_VSLLineC3Vect/1 -> Index Vector3/2
  LM_VSLLineC2Vect/1 -> Index Vector2/2
  Add1/1 -> Switch2/3
  Unit Delay1/1 -> Add1/2
  Product1/1 -> Add1/1, Switch2/1
  Switch2/1 -> LM_VSLBaseC2/1, Unit Delay1/1
  Switch3/1 -> Unit Delay2/1, LM_VSLBaseC3/1
  Relational Operator2/1 -> Switch8/2, Switch/2, Switch2/2, Switch3/2
  Product2/1 -> Switch3/1, Add2/1
  Unit Delay2/1 -> Add2/2
  Add2/1 -> Switch3/3
  Index Vector2/1 -> Product1/1
  LM_VSLMinQualityLineValid/1 -> Switch4/2
  Constant1/1 -> Switch4/3
  Index Vector4/1 -> Logical Operator1/1
  Switch1/1 -> Switch6/3
  Add3/1 -> Switch8/3
  Unit Delay3/1 -> Add3/2
  Product3/1 -> Add3/1, Switch8/1
  Switch8/1 -> Unit Delay3/1, Product4/2

== system PubIfDecisionLM_MDL/Subsystem2/LM_VSL/LM_VSLFntPath/LM_VSL_LineInfoEvalutaion/LM_VSL_BaseLinePCalc3/Subsystem/Switch Case Action Subsystem3/LM_VSLLineQualitySumCalc ==
  LM_VSLLineMinQualityIndex : Inport
  LM_VSLLineQualityVect : Inport  Port=2
  LM_VSLMinQualityLineValid : Inport  Port=3
  Diffnum : Inport  Port=4
  LM_VSLDiffValidIndex : Inport  Port=5
  Add : Sum
  Constant : Constant
  Constant1 : Constant  Value=0  OutDataTypeStr=single
  Constant2 : Constant  Value=0  OutDataTypeStr=single
  For Iterator : ForIterator  IterationLimit=4
  Index Vector : MultiPortSwitch  Inputs=1
  Index Vector1 : MultiPortSwitch  Inputs=1
  Logical Operator1 : Logic  Operator=NOT  AllPortsSameDT=off  OutDataTypeStr=boolean
  Relational Operator : RelationalOperator  Operator===  OutDataTypeStr=boolean  RndMeth=Nearest
  Relational Operator1 : RelationalOperator  Operator===  OutDataTypeStr=boolean  RndMeth=Nearest
  Switch{,1..3} (4 alike) : Switch  Criteria=u2 ~= 0
  Terminator : Terminator
  Unit Delay : UnitDelay  SampleTime=-1  HasFrameUpgradeWarning=on
  LM_VSLLineQualitySum : Outport
  wires:
  For Iterator/1 -> Relational Operator/1, Index Vector1/1, Relational Operator1/2, Index Vector/1
  Constant/1 -> Relational Operator/2
  Relational Operator/1 -> Switch/2
  LM_VSLLineMinQualityIndex/1 -> Relational Operator1/1
  Relational Operator1/1 -> Switch1/2
  LM_VSLLineQualityVect/1 -> Index Vector/2
  Index Vector/1 -> Switch2/1, Switch1/3
  Switch2/1 -> Switch1/1
  Switch3/1 -> Switch/1, Add/1
  Add/1 -> Switch/3
  Switch/1 -> Unit Delay/1, LM_VSLLineQualitySum/1  "LM_VSLLineQualitySum"
  Unit Delay/1 -> Add/2
  LM_VSLMinQualityLineValid/1 -> Switch2/2
  Constant1/1 -> Switch2/3
  Switch1/1 -> Switch3/3
  LM_VSLDiffValidIndex/1 -> Index Vector1/2
  Constant2/1 -> Switch3/1
  Index Vector1/1 -> Logical Operator1/1
  Logical Operator1/1 -> Switch3/2
  Diffnum/1 -> Terminator/1

== system PubIfDecisionLM_MDL/Subsystem2/LM_VSL/LM_VSLFntPath/LM_VSL_LineInfoEvalutaion/LM_VSL_LineInfoEvalutaion/LM_VSL_LineQualityEvalutaion/If Action Subsystem1/For Iterator Subsystem ==
  LM_VSLLineQualityVect : Inport
  Constant : Constant
  Constant1 : Constant  Value=0
  Constant2 : Constant  Value=255  OutDataTypeStr=uint8
  Constant3 : Constant  Value=0  OutDataTypeStr=uint8
  Constant4 : Constant  OutDataTypeStr=uint8
  For Iterator : ForIterator  IterationLimit=4
  Index Vector : MultiPortSwitch  Inputs=1
  Relational Operator : RelationalOperator  Operator===  OutDataTypeStr=boolean  RndMeth=Nearest
  Relational Operator1 : RelationalOperator  Operator===  OutDataTypeStr=boolean  RndMeth=Nearest
  Relational Operator2 : RelationalOperator  Operator=<  OutDataTypeStr=boolean  RndMeth=Nearest
  Switch{,1..2,4..5} (5 alike) : Switch  Criteria=u2 ~= 0
  Switch3 : Switch  Criteria=u2 ~= 0  OutDataTypeStr=int32
  Unit Delay : UnitDelay  SampleTime=-1  HasFrameUpgradeWarning=on
  Unit Delay1 : UnitDelay  SampleTime=-1  HasFrameUpgradeWarning=on
  LM_VSLLineMinQuality : Outport
  LM_VSLLineMinQualityIndex : Outport  Port=2
  wires:
  For Iterator/1 -> Relational Operator/1, Switch5/1, Index Vector/1
  LM_VSLLineQualityVect/1 -> Index Vector/2
  Constant/1 -> Relational Operator/2
  Relational Operator/1 -> Switch3/2, Switch/2
  Index Vector/1 -> Switch1/3, Relational Operator1/1
  Constant1/1 -> Relational Operator1/2
  Relational Operator1/1 -> Switch1/2, Switch4/2
  Constant2/1 -> Switch1/1
  Switch1/1 -> Switch/1, Switch2/1, Relational Operator2/1
  Unit Delay/1 -> Switch2/3, Relational Operator2/2
  Relational Operator2/1 -> Switch5/2, Switch2/2
  Switch/1 -> LM_VSLLineMinQuality/1, Unit Delay/1  "LM_VSLLineMinQuality"
  Switch2/1 -> Switch/3
  Constant3/1 -> Switch4/1
  Constant4/1 -> Switch4/3
  Switch4/1 -> Switch3/1
  Unit Delay1/1 -> Switch5/3
  Switch3/1 -> LM_VSLLineMinQualityIndex/1, Unit Delay1/1  "LM_VSLLineMinQualityIndex"
  Switch5/1 -> Switch3/3

== system PubIfDecisionLM_MDL/Subsystem2/LM_Fusion1/LM_FusRatioCalc/LM_Fusion_EO/LM_FusEVORatioCalc/LM_Fusion_FntPathK/LM_FusEOFntPath1/If Action Subsystem1/LM_FusEOFntPath1RatioCalc ==
  note: 当OTL第一段轨迹质量高于0.65，且车辆没有换道或转弯行为时，EML的质量为用车速查的修正值，否则EML质量修真值为0.95，即当第一段OTL质量不是很高时，EML的质量修正系数不能太小，适当提高EML占比
  vxvRefMs : Inport
  LM_FusEVOFntPath1EMLFac : Inport  Port=2
  LM_FusEVOFntPath1OTLFac : Inport  Port=3
  LM_EMLFntPath1Quality : Inport  Port=4
  LM_OTLFntPath1Qulity : Inport  Port=5
  Add1 : Sum
  Constant : Constant  Value=0.65  OutDataTypeStr=single
  Constant1 : Constant  Value=0.95  OutDataTypeStr=single
  Constant2 : Constant  Value=10  OutDataTypeStr=single
  Constant3 : Constant  Value=6  OutDataTypeStr=single
  Constant4 : Constant  Value=0.6  OutDataTypeStr=single
  Constant5 : Constant  Value=0.45  OutDataTypeStr=single
  Constant6 : Constant  OutDataTypeStr=single
  Constant7 : Constant  Value=0.6
  Divide : Product  Inputs=*/
  Divide2 : Product  Inputs=*/
  Logical Operator : Logic  AllPortsSameDT=off  OutDataTypeStr=boolean
  Logical Operator1 : Logic  AllPortsSameDT=off  OutDataTypeStr=boolean
  Max : MinMax  Function=max  Inputs=2
  Max1 : MinMax  Function=max  Inputs=2
  Product : Product
  Product2 : Product
  Relational Operator{,1..3} (4 alike) : RelationalOperator  OutDataTypeStr=boolean  RndMeth=Simplest
  Subtract : Sum  Inputs=+-
  Switch{,1..3} (4 alike) : Switch  Criteria=u2 ~= 0
  LM_FusEOFntPath1EMLK : Outport
  LM_FusEOFntPath1OTLK : Outport  Port=2
  wires:
  Divide2/1 -> Switch3/3
  Switch1/1 -> LM_FusEOFntPath1EMLK/1, Subtract/2  "LM_FusEOFntPath1EMLK"
  Add1/1 -> Divide/2, Divide2/2
  Product2/1 -> Add1/2, Divide2/1
  Product/1 -> Add1/1, Divide/1
  LM_OTLFntPath1Qulity/1 -> Product2/1, Relational Operator/1
  LM_FusEVOFntPath1OTLFac/1 -> Product2/2
  LM_EMLFntPath1Quality/1 -> Relational Operator3/1, Product/1
  LM_FusEVOFntPath1EMLFac/1 -> Switch/1
  Constant/1 -> Relational Operator/2
  Relational Operator/1 -> Switch/2
  Switch/1 -> Product/2
  Constant1/1 -> Switch/3
  vxvRefMs/1 -> Relational Operator2/1, Relational Operator1/1
  Constant2/1 -> Relational Operator1/2
  Logical Operator/1 -> Switch1/2
  Constant3/1 -> Relational Operator2/2
  Logical Operator1/1 -> Switch3/2, Switch2/2
  Constant4/1 -> Max/2
  Divide/1 -> Switch2/3, Max/1, Max1/1  "LM_FusEOFntPath1EMLK"
  Max/1 -> Switch1/1
  Switch2/1 -> Switch1/3
  Constant5/1 -> Max1/2
  Max1/1 -> Switch2/1
  Constant6/1 -> Subtract/1
  Subtract/1 -> Switch3/1
  Switch3/1 -> LM_FusEOFntPath1OTLK/1  "LM_FusEOFntPath1OTLK"
  Constant7/1 -> Relational Operator3/2
  Relational Operator3/1 -> Logical Operator1/1, Logical Operator/1
  Relational Operator1/1 -> Logical Operator/2
  Relational Operator2/1 -> Logical Operator1/2

== system PubIfDecisionLM_MDL/Subsystem2/LM_Fusion1/LM_FusRatioCalc/LM_Fusion_EO/LM_FusEVORatioCalc/LM_Fusion_FntPathK/LM_FusEOFntPath1/If Action Subsystem1/LM_FusEO_EMLFactor ==
  vxvRefMs : Inport
  1-D Lookup Table : Lookup_n-D  NumberOfTableDimensions=1  BreakpointsForDimension1=single([5,15,25,35,50]);  Table=[0.2,0.5,0.65,0.8,0.9]  InternalRulePriority=Speed  RndMeth=Simplest  InputSameDT=on
  LM_FusEVOFntPath1EMLFac : Outport
  wires:
  1-D Lookup Table/1 -> LM_FusEVOFntPath1EMLFac/1
  vxvRefMs/1 -> 1-D Lookup Table/1

== system PubIfDecisionLM_MDL/Subsystem2/LM_Fusion1/LM_FusRatioCalc/LM_Fusion_EO/LM_FusEVORatioCalc/LM_Fusion_FntPathK/LM_FusEOFntPath1/If Action Subsystem1/LM_FusEO_OTLFactor ==
  Constant : Constant  Value=0.65  OutDataTypeStr=single
  LM_FusEVOFntPath1OTLFac : Outport
  wires:
  Constant/1 -> LM_FusEVOFntPath1OTLFac/1

== system PubIfDecisionLM_MDL/Subsystem2/LM_Fusion1/LM_FusRatioCalc/LM_Fusion_EVO/LM_FusEVORatioCalc/LM_Fusion_FntPathK/LM_FusEVOFntPath1/If Action Subsystem1/LM_FusEVORatioCalc ==
  LM_FusEVOFntPath1EMLFac : Inport
  LM_FusEVOFntPath1VSLFac : Inport  Port=2
  LM_FusEVOFntPath1OTLFac : Inport  Port=3
  LM_VSLFntPath1Quality : Inport  Port=4
  LM_EMLFntPath1Quality : Inport  Port=5
  LM_OTLFntPath1Qulity : Inport  Port=6
  Add : Sum
  Add1 : Sum
  Divide : Product  Inputs=*/
  Divide1 : Product  Inputs=*/
  Divide2 : Product  Inputs=*/
  Product : Product
  Product1 : Product
  Product2 : Product
  LM_FusEVOFntPath1EMLK : Outport
  LM_FusEVOFntPath1VSLK : Outport  Port=2
  LM_FusEVOFntPath1OTLK : Outport  Port=3
  wires:
  LM_FusEVOFntPath1EMLFac/1 -> Product/2
  LM_EMLFntPath1Quality/1 -> Product/1
  LM_FusEVOFntPath1VSLFac/1 -> Product1/2
  LM_VSLFntPath1Quality/1 -> Product1/1
  LM_FusEVOFntPath1OTLFac/1 -> Product2/2
  LM_OTLFntPath1Qulity/1 -> Product2/1
  Product/1 -> Add/1, Divide/1
  Product1/1 -> Divide1/1, Add/2
  Add/1 -> Add1/1
  Product2/1 -> Divide2/1, Add1/2
  Add1/1 -> Divide2/2, Divide1/2, Divide/2
  Divide/1 -> LM_FusEVOFntPath1EMLK/1
  Divide1/1 -> LM_FusEVOFntPath1VSLK/1
  Divide2/1 -> LM_FusEVOFntPath1OTLK/1

== system PubIfDecisionLM_MDL/Subsystem2/LM_Fusion1/LM_FusRatioCalc/LM_Fusion_EVO/LM_FusEVORatioCalc/LM_Fusion_FntPathK/LM_FusEVOFntPath1/If Action Subsystem1/LM_FusEVO_EMLFactor ==
  vxvRefMs : Inport
  DIR_LC2LeValid : Inport  Port=2
  DIR_LC2RigValid : Inport  Port=3
  1-D Lookup Table : Lookup_n-D  NumberOfTableDimensions=1  BreakpointsForDimension1=single([5,15,25,35,50]);  Table=[0.2,0.5,0.65,0.8,0.9]  InternalRulePriority=Speed  RndMeth=Simplest  InputSameDT=on
  Constant : Constant  Value=0.5  OutDataTypeStr=single
  Logical Operator : Logic  Operator=OR  AllPortsSameDT=off  OutDataTypeStr=boolean
  Switch : Switch  Criteria=u2 ~= 0
  LM_FusEVOFntPath1EMLFac : Outport
  wires:
  vxvRefMs/1 -> 1-D Lookup Table/1
  1-D Lookup Table/1 -> Switch/3
  DIR_LC2LeValid/1 -> Logical Operator/1
  DIR_LC2RigValid/1 -> Logical Operator/2
  Logical Operator/1 -> Switch/2
  Constant/1 -> Switch/1
  Switch/1 -> LM_FusEVOFntPath1EMLFac/1

== system PubIfDecisionLM_MDL/Subsystem2/LM_Fusion1/LM_FusRatioCalc/LM_Fusion_EVO/LM_FusEVORatioCalc/LM_Fusion_FntPathK/LM_FusEVOFntPath1/If Action Subsystem1/LM_FusEVO_OTLFactor ==
  DIR_LC2LeValid : Inport
  DIR_LC2RigValid : Inport  Port=2
  Constant : Constant  Value=P_LM_FusEVOPath1OTLFacNLC  OutDataTypeStr=single
  Constant1 : Constant  Value=0  OutDataTypeStr=single
  Logical Operator : Logic  Operator=OR  AllPortsSameDT=off  OutDataTypeStr=boolean
  Switch : Switch  Criteria=u2 ~= 0
  LM_FusEVOFntPath1OTLFac : Outport
  wires:
  DIR_LC2LeValid/1 -> Logical Operator/1
  Constant1/1 -> Switch/1
  Constant/1 -> Switch/3
  Logical Operator/1 -> Switch/2
  DIR_LC2RigValid/1 -> Logical Operator/2
  Switch/1 -> LM_FusEVOFntPath1OTLFac/1

== system PubIfDecisionLM_MDL/Subsystem2/LM_Fusion1/LM_FusRatioCalc/LM_Fusion_EVO/LM_FusEVORatioCalc/LM_Fusion_FntPathK/LM_FusEVOFntPath1/If Action Subsystem1/LM_FusEVO_VSLFactor ==
  Constant : Constant  OutDataTypeStr=single
  LM_FusEVOFntPath1VSLFac : Outport
  wires:
  Constant/1 -> LM_FusEVOFntPath1VSLFac/1

== system PubIfDecisionLM_MDL/Subsystem2/LM_Fusion1/LM_FusRatioCalc/LM_Fusion_EVO/LM_FusEVORatioCalc/LM_Fusion_FntPathK/LM_FusEVOFntPath2/If Action Subsystem1/LM_FusEVO_EMLFactor ==
  vxvRefMs : Inport
  DIR_LC2LeValid : Inport  Port=2
  DIR_LC2RigValid : Inport  Port=3
  1-D Lookup Table : Lookup_n-D  NumberOfTableDimensions=1  BreakpointsForDimension1=single([5,15,25,35,50]);  Table=[0.1,0.3,0.45,0.6,0.75]  InternalRulePriority=Speed  RndMeth=Simplest  InputSameDT=on
  Constant : Constant  Value=0.3  OutDataTypeStr=single
  Logical Operator : Logic  Operator=OR  AllPortsSameDT=off  OutDataTypeStr=boolean
  Switch : Switch  Criteria=u2 ~= 0
  LM_FusEVOFntPath2EMLFac : Outport
  wires:
  Switch/1 -> LM_FusEVOFntPath2EMLFac/1  "LM_FusEVOFntPath2EMLFac"
  Constant/1 -> Switch/1
  Logical Operator/1 -> Switch/2
  DIR_LC2RigValid/1 -> Logical Operator/2
  DIR_LC2LeValid/1 -> Logical Operator/1
  1-D Lookup Table/1 -> Switch/3
  vxvRefMs/1 -> 1-D Lookup Table/1

== system PubIfDecisionLM_MDL/Subsystem2/LM_Fusion1/LM_FusRatioCalc/LM_Fusion_EVO/LM_FusEVORatioCalc/LM_Fusion_FntPathK/LM_FusEVOFntPath2/If Action Subsystem1/LM_FusEVO_OTLFactor ==
  DIR_LC2LeValid : Inport
  DIR_LC2RigValid : Inport  Port=2
  Constant : Constant  Value=0.85  OutDataTypeStr=single
  Constant1 : Constant  Value=0  OutDataTypeStr=single
  Logical Operator : Logic  Operator=OR  AllPortsSameDT=off  OutDataTypeStr=boolean
  Switch : Switch  Criteria=u2 ~= 0
  LM_FusEVOFntPath2OTLFac : Outport
  wires:
  Switch/1 -> LM_FusEVOFntPath2OTLFac/1
  DIR_LC2RigValid/1 -> Logical Operator/2
  Logical Operator/1 -> Switch/2
  Constant/1 -> Switch/3
  Constant1/1 -> Switch/1
  DIR_LC2LeValid/1 -> Logical Operator/1

== system PubIfDecisionLM_MDL/Subsystem2/LM_Fusion1/LM_FusRatioCalc/LM_Fusion_EVO/LM_FusEVORatioCalc/LM_Fusion_FntPathK/LM_FusEVOFntPath2/If Action Subsystem1/LM_FusEVO_VSLFactor ==
  Constant : Constant  Value=0.95  OutDataTypeStr=single
  LM_FusEVOFntPath2VSLFac : Outport
  wires:
  Constant/1 -> LM_FusEVOFntPath2VSLFac/1

== system PubIfDecisionLM_MDL/Subsystem2/LM_Fusion1/LM_FusRatioCalc/LM_Fusion_EVO/LM_FusEVORatioCalc/LM_Fusion_FntPathK/LM_FusEVOFntPath2/If Action Subsystem1/Subsystem ==
  LM_FusEVOFntPath2EMLFac : Inport
  LM_FusEVOFntPath2VSLFac : Inport  Port=2
  LM_FusEVOFntPath2OTLFac : Inport  Port=3
  LM_EMLFntPath2Quality : Inport  Port=4
  LM_VSLFntPath2Quality : Inport  Port=5
  LM_OTLFntPath2Qulity : Inport  Port=6
  Add : Sum
  Add1 : Sum
  Compare To Zero : simulink/Logic and Bit Operations/Compare To Zero  relop===  OutDataTypeStr=boolean
  Constant : Constant  Value=0.000001  OutDataTypeStr=single
  Divide : Product  Inputs=*/
  Divide1 : Product  Inputs=*/
  Divide2 : Product  Inputs=*/
  Product : Product
  Product1 : Product
  Product2 : Product
  Switch : Switch  Criteria=u2 ~= 0
  LM_FusEVOFntPath2EMLK : Outport
  LM_FusEVOFntPath2VSLK : Outport  Port=2
  LM_FusEVOFntPath2OTLK : Outport  Port=3
  wires:
  Divide1/1 -> LM_FusEVOFntPath2VSLK/1  "LM_FusEVOFntPath2VSLK"
  LM_FusEVOFntPath2EMLFac/1 -> Product/2
  Product1/1 -> Divide1/1, Add/2
  LM_VSLFntPath2Quality/1 -> Product1/1
  Product2/1 -> Divide2/1, Add1/2
  LM_EMLFntPath2Quality/1 -> Product/1
  Switch/1 -> Divide2/2, Divide1/2, Divide/2
  Product/1 -> Divide/1, Add/1
  LM_OTLFntPath2Qulity/1 -> Product2/1
  Divide/1 -> LM_FusEVOFntPath2EMLK/1  "LM_FusEVOFntPath2EMLK"
  LM_FusEVOFntPath2VSLFac/1 -> Product1/2
  Add/1 -> Add1/1
  LM_FusEVOFntPath2OTLFac/1 -> Product2/2
  Divide2/1 -> LM_FusEVOFntPath2OTLK/1  "LM_FusEVOFntPath2OTLK"
  Add1/1 -> Switch/3, Compare To Zero/1
  Compare To Zero/1 -> Switch/2
  Constant/1 -> Switch/1

== system PubIfDecisionLM_MDL/Subsystem2/LM_Fusion1/LM_FusRatioCalc/LM_Fusion_EVO/LM_FusEVORatioCalc/LM_Fusion_FntPathK/LM_FusEVOFntPath3/If Action Subsystem1/LM_FusEVO_EMLFactor ==
  vxvRefMs : Inport
  DIR_LC2LeValid : Inport  Port=2
  DIR_LC2RigValid : Inport  Port=3
  1-D Lookup Table : Lookup_n-D  NumberOfTableDimensions=1  BreakpointsForDimension1=single([5,15,25,35,50]);  Table=[0.05,0.15,0.25,0.45,0.55]  InternalRulePriority=Speed  RndMeth=Simplest  InputSameDT=on
  Constant : Constant  Value=0.1  OutDataTypeStr=single
  Logical Operator : Logic  Operator=OR  AllPortsSameDT=off  OutDataTypeStr=boolean
  Switch : Switch  Criteria=u2 ~= 0
  LM_FusEVOFntPath3EMLFac : Outport
  wires:
  vxvRefMs/1 -> 1-D Lookup Table/1
  1-D Lookup Table/1 -> Switch/3
  DIR_LC2LeValid/1 -> Logical Operator/1
  DIR_LC2RigValid/1 -> Logical Operator/2
  Logical Operator/1 -> Switch/2
  Constant/1 -> Switch/1
  Switch/1 -> LM_FusEVOFntPath3EMLFac/1  "LM_FusEVOFntPath3EMLFac"

== system PubIfDecisionLM_MDL/Subsystem2/LM_Fusion1/LM_FusRatioCalc/LM_Fusion_EVO/LM_FusEVORatioCalc/LM_Fusion_FntPathK/LM_FusEVOFntPath3/If Action Subsystem1/LM_FusEVO_OTLFactor ==
  DIR_LC2LeValid : Inport
  DIR_LC2RigValid : Inport  Port=2
  Constant : Constant  Value=0.75  OutDataTypeStr=single
  Constant1 : Constant  Value=0  OutDataTypeStr=single
  Logical Operator : Logic  Operator=OR  AllPortsSameDT=off  OutDataTypeStr=boolean
  Switch : Switch  Criteria=u2 ~= 0
  LM_FusEVOFntPath3OTLFac : Outport
  wires:
  DIR_LC2LeValid/1 -> Logical Operator/1
  Constant1/1 -> Switch/1
  Constant/1 -> Switch/3
  Logical Operator/1 -> Switch/2
  DIR_LC2RigValid/1 -> Logical Operator/2
  Switch/1 -> LM_FusEVOFntPath3OTLFac/1

== system PubIfDecisionLM_MDL/Subsystem2/LM_Fusion1/LM_FusRatioCalc/LM_Fusion_EVO/LM_FusEVORatioCalc/LM_Fusion_FntPathK/LM_FusEVOFntPath3/If Action Subsystem1/LM_FusEVO_VSLFactor ==
  Constant : Constant  Value=0.95  OutDataTypeStr=single
  LM_FusEVOFntPath3VSLFac : Outport
  wires:
  Constant/1 -> LM_FusEVOFntPath3VSLFac/1
